simulink model "simF16_lpvplant_unmatched"  (R2020a)
settings: Solver=ode14x  StartTime=0  StopTime=sim_t  FixedStep=Ts  RelTol=1e-3  EnableMultiTasking=on
values from neighbouring files (symbols this model uses):
  adapt_gain_no_Bm = -inv(Phi)*Mat_expm    [main_f16.m]
  Ap0 = [-0.965786131048  0.940676857343; -3.44113853073  -1.30180201506]    [lpv_model.mat]    (also in parameters_twoparas_ss_large_omega_range.mat)
  Ap1 = [-0.695446741137  -0.0219021350224; -2.98749239517  -0.883673052084]    [lpv_model.mat]    (also in parameters_twoparas_ss_large_omega_range.mat)
  Ap2 = [-0.00376589285085  -0.000767161245953; 0.0864223450734  -0.00373090940113]    [lpv_model.mat]    (also in parameters_twoparas_ss_large_omega_range.mat)
  Bp0 = [-0.00202220767716 -0.26458627897]    [lpv_model.mat]    (also in parameters_twoparas_ss_large_omega_range.mat)
  Bp1 = [-0.00144075289053 -0.241352628281]    [lpv_model.mat]    (also in parameters_twoparas_ss_large_omega_range.mat)
  Bp2 = [-6.1325666296e-07 -0.000135209280723]    [lpv_model.mat]    (also in parameters_twoparas_ss_large_omega_range.mat)
  Cp = [1 0]    [lpv_model.mat]    (also in parameters_twoparas_ss_large_omega_range.mat)
  enable_L1 = 1    [main_f16.m]
  enable_um_dist_comp = 1    [main_f16.m]
  L = [-1.0529546208e-07 9.01402394984e-07 -6.3448246624e-08 3.15977865752e-07 2.28928663113e-09 -4.32057794956e-09]    [parameters_twoparas_ss_large_omega_range.mat]
  opt =     [unmatched_comp_filter.mat]
  r2d = 180/pi    (= 57.2957795131)    [main_f16.m]
  sample_time = Ts    (= 0.001)    [main_f16.m]
  Ts = 1e-3    (= 0.001)    [main_f16.m]
  unknown_input_gain = .7    (= 0.7)    [main_f16.m]
  X = [4.80336810738e-09 -1.50779531784e-08 -1.50779531784e-08 7.69063603425e-08 2.19210658353e-09 -1.15520629836e-08 -1.15520629836e-08 6.7948487849e-08 9.47019033424e-11 -1.37129742327e-10 -1.37129742327e-10 2.78905243689e-10]    [parameters_twoparas_ss_large_omega_range.mat]
undefined symbols (not defined in the file or in its folder): C_den, C_num
settings Model: ExtModeAutoUpdateStatusClock=off  Creator=keviczky  LastModifiedBy=Boran
settings DataIOCC: Decimation=50  SaveFormat=Array  SignalLoggingSaveFormat=ModelDataLogs  ReturnWorkspaceOutputs=off  SignalLoggingName=sigsOut
settings OptimizationCC: BooleanDataType=off
settings DebuggingCC: AlgebraicLoopMsg=error  SaveWithParameterizedLinksMsg=none  UnderspecifiedInitializationDetection=Classic  MergeDetectMultiDrivingBlocksExec=none  SignalResolutionControl=TryResolveAllWithWarning  MultiTaskDSMMsg=warning  MultiTaskCondExecSysMsg=none  ArithmeticOperatorsInVariantConditions=warning
settings HardwareCC: ProdBitPerPointer=32  ProdBitPerSizeT=32  ProdBitPerPtrDiffT=32  ProdLargestAtomicFloat=None  ProdIntDivRoundTo=Undefined  ProdEndianess=Unspecified  ProdWordSize=32  ProdHWDeviceType=32-bit Generic  TargetUnknown=on
settings ModelReferenceCC: PropagateSignalLabelsOutOfModel=off
settings SFSimCC: CustomCodeUndefinedFunction=UseInterfaceOnly
settings GRTTargetCC: CombineOutputUpdateFcns=off  GRTInterface=on
settings ConfigComp: CovMetricSettings=dw  CovHtmlReporting=on  CovSaveCumulativeToWorkspaceVar=on  CovSaveSingleToWorkspaceVar=on

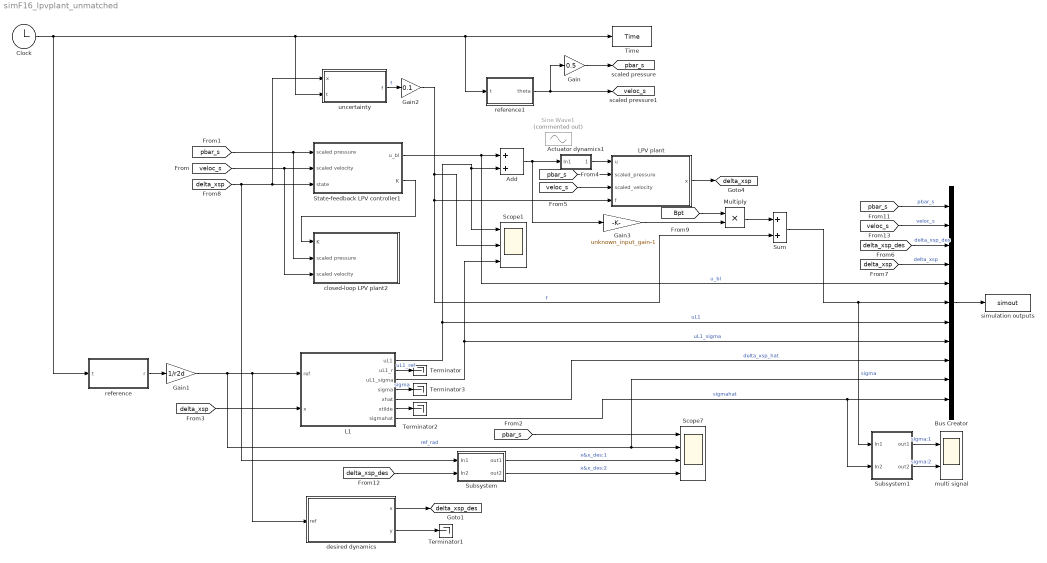
== system simF16_lpvplant_unmatched ==
  " LPV plant" : Subsystem
  Actuator dynamics1 : Subsystem
  Add : Sum
  Bus Creator : BusCreator  Inputs=11
  Clock : Clock
      settings: Decimation=50
  Gain : Gain  Gain=0.5
  Gain1 : Gain  Gain=1/r2d
  Gain2 : Gain  Gain=0.1
  Gain3 : Gain  Gain=unknown_input_gain-1
  L1 : Subsystem
  Multiply : Product
  Scope1 : Scope  NumInputPorts=3
  Scope7 : Scope  NumInputPorts=4
  Sine Wave1 : Sin  Commented=on  Frequency=2*pi*0.2  SampleTime=0
  State-feedback LPV controller1 : Subsystem
  Subsystem : Subsystem
  Subsystem1 : Subsystem
  Sum : Sum
  Terminator{,1..3} (4 alike) : Terminator
  Time : ToWorkspace  VariableName=Time  SampleTime=-1
  closed-loop LPV plant2 : Subsystem
  desired dynamics : Subsystem
  "multi signal " : Scope  NumInputPorts=2
  reference : MATLAB Function  TreatAsAtomicUnit=on
  reference1 : MATLAB Function  TreatAsAtomicUnit=on
  simulation outputs : ToWorkspace  VariableName=simout  SaveFormat=Timeseries  SampleTime=-1
  uncertainty : MATLAB Function  TreatAsAtomicUnit=on
  tag scope: delta_xsp=global, delta_xsp_des=global, pbar_s=global, veloc_s=global
  wires:
  [veloc_s] -> closed-loop LPV plant2/3(scaled velocity), State-feedback LPV controller1/2(scaled velocity)
  [pbar_s] -> closed-loop LPV plant2/2(scaled pressure), State-feedback LPV controller1/1(scaled pressure)
  State-feedback LPV controller1/2(K) -> closed-loop LPV plant2/1(K)
  State-feedback LPV controller1/1(u_bl) -> Bus Creator/5, Add/1  "u_bl"
  reference/1(r) -> Gain1/1
  Gain/1 -> [pbar_s]
  [pbar_s] -> " LPV plant"/2(scaled_pressure)
  " LPV plant"/1(x) -> [delta_xsp]
  [pbar_s] -> Scope7/1
  [delta_xsp] -> L1/2(x)
  L1/1(uL1) -> Scope1/1, Add/2, Bus Creator/7  "uL1"
  Add/1 -> Gain3/1, Actuator dynamics1/1(In1)
  Clock/1 -> reference1/1(t), Time/1, uncertainty/2(t), reference/1(t)
  L1/3(uL1_sigma) -> Scope1/3, Bus Creator/8  "uL1_sigma"
  reference1/1(theta) -> Gain/1, [veloc_s]
  [delta_xsp] -> uncertainty/1(x), State-feedback LPV controller1/3(state), Subsystem/1(In1)
  [veloc_s] -> " LPV plant"/3(scaled_velocity)
  Bus Creator/1 -> simulation outputs/1
  L1/2(uL1_r) -> Terminator/1  "uL1_ref"
  desired dynamics/1(x) -> [delta_xsp_des]
  [delta_xsp_des] -> Subsystem/2(In2)
  Subsystem/1(out1) -> Scope7/3  "x&x_des:1"
  Subsystem/2(out2) -> Scope7/4  "x&x_des:2"
  desired dynamics/2(y) -> Terminator1/1
  [pbar_s] -> Bus Creator/1  "pbar_s"
  [veloc_s] -> Bus Creator/2  "veloc_s"
  [delta_xsp_des] -> Bus Creator/3  "delta_xsp_des"
  [delta_xsp] -> Bus Creator/4  "delta_xsp"
  uncertainty/1(f) -> Gain2/1  "f"
  L1/5(xhat) -> Bus Creator/9  "delta_xsp_hat"
  Gain1/1 -> Bus Creator/10, Scope7/2, L1/1(ref), desired dynamics/1(ref)  "ref_rad"
  L1/6(xtilde) -> Terminator2/1
  Gain2/1 -> " LPV plant"/4(f), Sum/2, Scope1/2  "f"
  L1/4(sigma) -> Terminator3/1  "sigma"
  L1/7(sigmahat) -> Subsystem1/2(In2), Bus Creator/11  "sigmahat"
  [Bpt] -> Multiply/1
  Gain3/1 -> Multiply/2
  Multiply/1 -> Sum/1
  Sum/1 -> Subsystem1/1(In1), Bus Creator/6  "sigma"
  Subsystem1/1(out1) -> "multi signal "/1  "sigma:1"
  Subsystem1/2(out2) -> "multi signal "/2  "sigma:2"
  Actuator dynamics1/1(Out1) -> " LPV plant"/1(u)

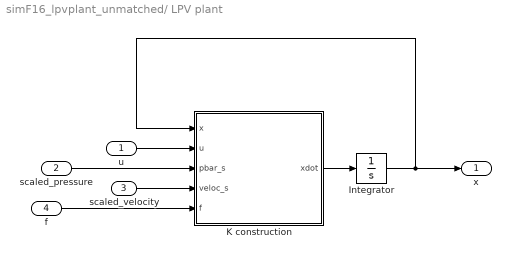
== system simF16_lpvplant_unmatched/ LPV plant ==
  u : Inport
  scaled_pressure : Inport  Port=2
  scaled_velocity : Inport  Port=3
  f : Inport  Port=4
  Integrator : Integrator
  K construction : MATLAB Function  TreatAsAtomicUnit=on
  x : Outport  VectorParamsAs1DForOutWhenUnconnected=off
  wires:
  scaled_pressure/1 -> K construction/3(pbar_s)
  u/1 -> K construction/2(u)
  K construction/1(xdot) -> Integrator/1
  Integrator/1 -> x/1, K construction/1(x)
  scaled_velocity/1 -> K construction/4(veloc_s)
  f/1 -> K construction/5(f)

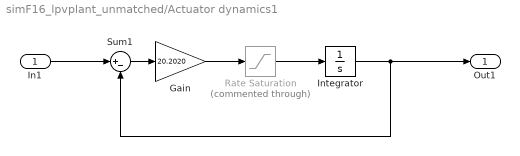
== system simF16_lpvplant_unmatched/Actuator dynamics1 ==
  In1 : Inport
  Gain : Gain  Gain=20.2020  SaturateOnIntegerOverflow=on  OutDataTypeStr=Inherit: Same as input  ParamDataTypeStr=Inherit: Same as input
  Integrator : Integrator  UpperSaturationLimit=25  LowerSaturationLimit=-25
  Rate Saturation : Saturate  Commented=through  UpperLimit=60  LowerLimit=-60
  Sum1 : Sum  Inputs=|+-  InputSameDT=on  SaturateOnIntegerOverflow=on  OutDataTypeStr=Inherit: Same as first input
  Out1 : Outport  VectorParamsAs1DForOutWhenUnconnected=off
  wires:
  Sum1/1 -> Gain/1
  Gain/1 -> Rate Saturation/1
  Integrator/1 -> Out1/1, Sum1/2
  Rate Saturation/1 -> Integrator/1
  In1/1 -> Sum1/1

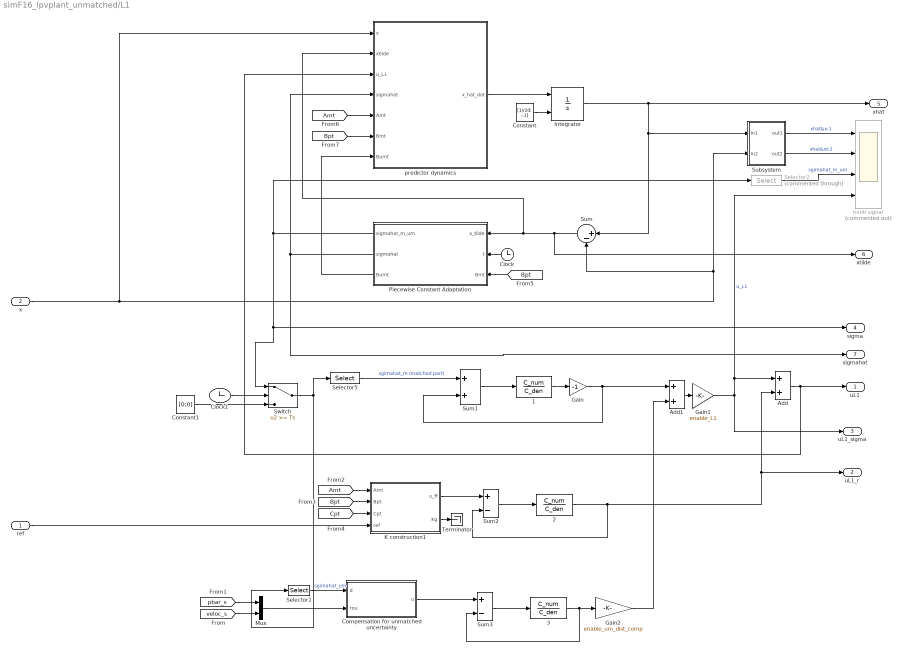
== system simF16_lpvplant_unmatched/L1 ==
  ref : Inport
  x : Inport  Port=2
  " 1" : TransferFcn  Numerator=C_num  Denominator=C_den
  " 2" : TransferFcn  Numerator=C_num  Denominator=C_den
  " 3" : TransferFcn  Numerator=C_num  Denominator=C_den
  Add : Sum
  Add1 : Sum
  Clock : Clock
  Clock1 : Clock
      settings: Decimation=50
  Compensation for unmatched uncertainty : Subsystem
  Constant : Constant  Value=[1/r2d; -.1]
  Constant1 : Constant  Value=[0;0]
  Gain : Gain  Gain=-1
  Gain1 : Gain  Gain=enable_L1
  Gain2 : Gain  Gain=enable_um_dist_comp
  Integrator : Integrator  InitialConditionSource=external
  K construction1 : MATLAB Function  TreatAsAtomicUnit=on
  Mux : Mux  Inputs=2
  Piecewise Constant Adaptation : MATLAB Function  TreatAsAtomicUnit=on
  Selector1 : Selector  InputPortWidth=2  IndexOptions=Index vector (dialog)  Indices=2  OutputSizes=1
  Selector2 : Selector  Commented=through  InputPortWidth=2  IndexOptions=Index vector (dialog)  Indices=[1]  OutputSizes=1
  Selector5 : Selector  InputPortWidth=2  IndexOptions=Index vector (dialog)  Indices=[1]  OutputSizes=1
  Subsystem : Subsystem
  Sum : Sum  Inputs=|+-
  Sum1 : Sum
  Sum2 : Sum  Inputs=+-
  Sum3 : Sum  Inputs=+-
  Switch : Switch  Threshold=Ts
  Terminator : Terminator
  "multi signal " : Scope  Commented=on  NumInputPorts=4
  predictor dynamics : MATLAB Function  TreatAsAtomicUnit=on
  uL1 : Outport  VectorParamsAs1DForOutWhenUnconnected=off
  uL1_r : Outport  Port=2  VectorParamsAs1DForOutWhenUnconnected=off
  uL1_sigma : Outport  Port=3  VectorParamsAs1DForOutWhenUnconnected=off
  sigma : Outport  Port=4  VectorParamsAs1DForOutWhenUnconnected=off
  xhat : Outport  Port=5  VectorParamsAs1DForOutWhenUnconnected=off
  xtilde : Outport  Port=6  VectorParamsAs1DForOutWhenUnconnected=off
  sigmahat : Outport  Port=7  VectorParamsAs1DForOutWhenUnconnected=off
  wires:
  Constant/1 -> Integrator/2
  predictor dynamics/1(x_hat_dot) -> Integrator/1
  Integrator/1 -> xhat/1, Sum/1, Subsystem/1(In1)
  Clock/1 -> Piecewise Constant Adaptation/2(t)
  x/1 -> Subsystem/2(In2), Sum/2, predictor dynamics/1(x)
  Piecewise Constant Adaptation/1(sigmahat_m_um) -> Switch/1, sigma/1, Selector2/1
  Selector2/1 -> "multi signal "/3  "sgimahat_m_um"
  Gain/1 -> Add1/1, Sum1/2
  " 1"/1 -> Gain/1
  [Cpt] -> K construction1/3(Cpt)
  [Bpt] -> K construction1/2(Bpt)
  ref/1 -> K construction1/4(ref)
  [Amt] -> K construction1/1(Amt)
  [Bpt] -> Piecewise Constant Adaptation/3(Bmt)
  [Amt] -> predictor dynamics/5(Amt)
  [Bpt] -> predictor dynamics/6(Bmt)
  Sum/1 -> xtilde/1, predictor dynamics/2(xtilde), Piecewise Constant Adaptation/1(x_tilde)
  Selector5/1 -> Sum1/1  "sgimahat_m (matched part)"
  Sum1/1 -> " 1"/1
  Piecewise Constant Adaptation/3(Bumt) -> predictor dynamics/7(Bumt)
  Sum2/1 -> " 2"/1
  " 2"/1 -> Sum2/2, Add/2, uL1_r/1
  Subsystem/1(out1) -> "multi signal "/1  "xhat&x:1"
  Subsystem/2(out2) -> "multi signal "/2  "xhat&xt:2"
  Add/1 -> predictor dynamics/3(u_L1), uL1/1
  K construction1/2(Kg) -> Terminator/1
  Gain1/1 -> uL1_sigma/1, Add/1, "multi signal "/4  "u_L1"
  Selector1/1 -> Compensation for unmatched uncertainty/1(d)  "sgimahat_um"
  [pbar_s] -> Mux/1
  [veloc_s] -> Mux/2
  Mux/1 -> Compensation for unmatched uncertainty/2(rou)
  " 3"/1 -> Gain2/1, Sum3/2
  Sum3/1 -> " 3"/1
  Compensation for unmatched uncertainty/1(u) -> Sum3/1
  Gain2/1 -> Add1/2
  Piecewise Constant Adaptation/2(sigmahat) -> predictor dynamics/4(sigmahat), sigmahat/1
  Add1/1 -> Gain1/1
  Switch/1 -> Selector1/1, Selector5/1
  Constant1/1 -> Switch/3
  Clock1/1 -> Switch/2
  K construction1/1(u_ff) -> Sum2/1

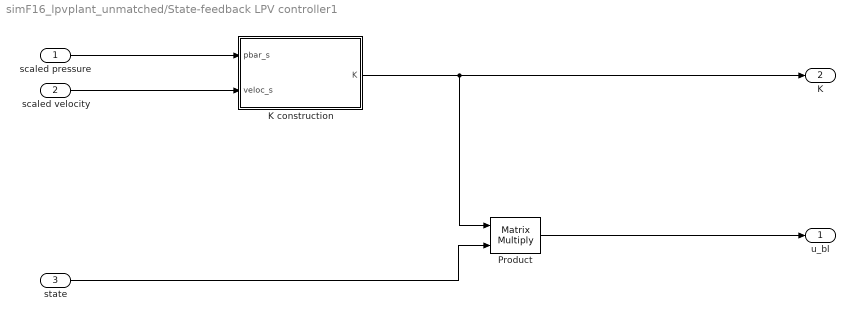
== system simF16_lpvplant_unmatched/State-feedback LPV controller1 ==
  scaled pressure : Inport
  scaled velocity : Inport  Port=2
  state : Inport  Port=3
  K construction : MATLAB Function  TreatAsAtomicUnit=on
  Product : Product  Multiplication=Matrix(*)
  u_bl : Outport  VectorParamsAs1DForOutWhenUnconnected=off
  K : Outport  Port=2  VectorParamsAs1DForOutWhenUnconnected=off
  wires:
  scaled pressure/1 -> K construction/1(pbar_s)
  K construction/1(K) -> Product/1, K/1
  state/1 -> Product/2
  Product/1 -> u_bl/1
  scaled velocity/1 -> K construction/2(veloc_s)

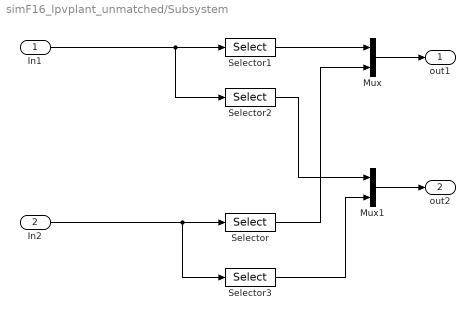
== system simF16_lpvplant_unmatched/Subsystem ==
  In1 : Inport
  In2 : Inport  Port=2
  Mux : Mux  Inputs=2
  Mux1 : Mux  Inputs=2
  Selector : Selector  InputPortWidth=2  IndexOptions=Index vector (dialog)  Indices=[1]  OutputSizes=1
  Selector1 : Selector  InputPortWidth=2  IndexOptions=Index vector (dialog)  Indices=[1]  OutputSizes=1
  Selector2 : Selector  InputPortWidth=2  IndexOptions=Index vector (dialog)  Indices=2  OutputSizes=1
  Selector3 : Selector  InputPortWidth=2  IndexOptions=Index vector (dialog)  Indices=2  OutputSizes=1
  out1 : Outport  VectorParamsAs1DForOutWhenUnconnected=off
  out2 : Outport  Port=2  VectorParamsAs1DForOutWhenUnconnected=off
  wires:
  In1/1 -> Selector2/1, Selector1/1
  In2/1 -> Selector3/1, Selector/1
  Selector/1 -> Mux/2
  Selector1/1 -> Mux/1
  Mux/1 -> out1/1
  Selector2/1 -> Mux1/1
  Selector3/1 -> Mux1/2
  Mux1/1 -> out2/1

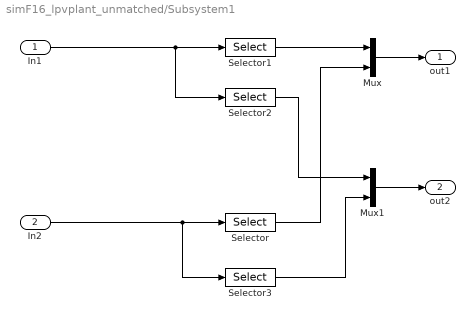
== system simF16_lpvplant_unmatched/Subsystem1 ==
  In1 : Inport
  In2 : Inport  Port=2
  Mux : Mux  Inputs=2
  Mux1 : Mux  Inputs=2
  Selector : Selector  InputPortWidth=2  IndexOptions=Index vector (dialog)  Indices=[1]  OutputSizes=1
  Selector1 : Selector  InputPortWidth=2  IndexOptions=Index vector (dialog)  Indices=[1]  OutputSizes=1
  Selector2 : Selector  InputPortWidth=2  IndexOptions=Index vector (dialog)  Indices=2  OutputSizes=1
  Selector3 : Selector  InputPortWidth=2  IndexOptions=Index vector (dialog)  Indices=2  OutputSizes=1
  out1 : Outport  VectorParamsAs1DForOutWhenUnconnected=off
  out2 : Outport  Port=2  VectorParamsAs1DForOutWhenUnconnected=off
  wires:
  In1/1 -> Selector2/1, Selector1/1
  In2/1 -> Selector3/1, Selector/1
  Selector/1 -> Mux/2
  Selector1/1 -> Mux/1
  Mux/1 -> out1/1
  Selector2/1 -> Mux1/1
  Selector3/1 -> Mux1/2
  Mux1/1 -> out2/1

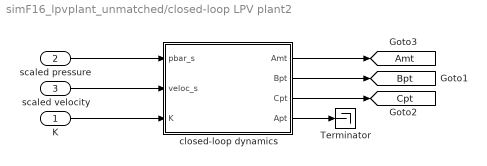
== system simF16_lpvplant_unmatched/closed-loop LPV plant2 ==
  K : Inport
  scaled pressure : Inport  Port=2
  scaled velocity : Inport  Port=3
  Terminator : Terminator
  closed-loop dynamics : MATLAB Function  TreatAsAtomicUnit=on
  tag scope: Amt=global, Bpt=global, Cpt=global
  wires:
  scaled pressure/1 -> closed-loop dynamics/1(pbar_s)
  K/1 -> closed-loop dynamics/3(K)
  closed-loop dynamics/3(Cpt) -> [Cpt]
  scaled velocity/1 -> closed-loop dynamics/2(veloc_s)
  closed-loop dynamics/1(Amt) -> [Amt]
  closed-loop dynamics/2(Bpt) -> [Bpt]
  closed-loop dynamics/4(Apt) -> Terminator/1

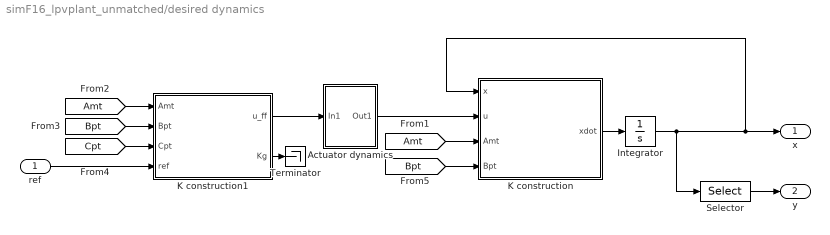
== system simF16_lpvplant_unmatched/desired dynamics ==
  ref : Inport
  Actuator dynamics : Subsystem
  Integrator : Integrator
  K construction : MATLAB Function  TreatAsAtomicUnit=on
  K construction1 : MATLAB Function  TreatAsAtomicUnit=on
  Selector : Selector  InputPortWidth=2  IndexOptions=Index vector (dialog)  Indices=1  OutputSizes=1
  Terminator : Terminator
  x : Outport  VectorParamsAs1DForOutWhenUnconnected=off
  y : Outport  Port=2  VectorParamsAs1DForOutWhenUnconnected=off
  wires:
  K construction1/2(Kg) -> Terminator/1
  [Bpt] -> K construction1/2(Bpt)
  [Amt] -> K construction1/1(Amt)
  K construction1/1(u_ff) -> Actuator dynamics/1(In1)
  ref/1 -> K construction1/4(ref)
  [Cpt] -> K construction1/3(Cpt)
  Integrator/1 -> Selector/1, x/1, K construction/1(x)
  K construction/1(xdot) -> Integrator/1
  [Amt] -> K construction/3(Amt)
  [Bpt] -> K construction/4(Bpt)
  Selector/1 -> y/1
  Actuator dynamics/1(Out1) -> K construction/2(u)

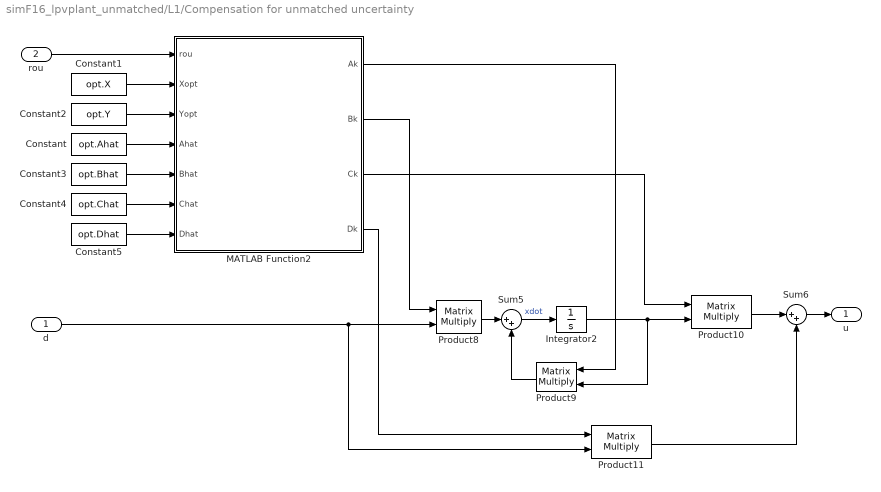
== system simF16_lpvplant_unmatched/L1/Compensation for unmatched uncertainty ==
  d : Inport
  rou : Inport  Port=2
  Constant : Constant  Value=opt.Ahat  VectorParams1D=off
  Constant1 : Constant  Value=opt.X  VectorParams1D=off
  Constant2 : Constant  Value=opt.Y  VectorParams1D=off
  Constant3 : Constant  Value=opt.Bhat  VectorParams1D=off
  Constant4 : Constant  Value=opt.Chat  VectorParams1D=off
  Constant5 : Constant  Value=opt.Dhat  VectorParams1D=off
  Integrator2 : Integrator
  MATLAB Function2 : MATLAB Function  TreatAsAtomicUnit=on
  Product{8..11} (4 alike) : Product  Multiplication=Matrix(*)
  Sum5 : Sum  Inputs=|++
  Sum6 : Sum  Inputs=|++
  u : Outport  VectorParamsAs1DForOutWhenUnconnected=off
  wires:
  d/1 -> Product8/2, Product11/2
  Sum5/1 -> Integrator2/1  "xdot"
  Product8/1 -> Sum5/1
  Product11/1 -> Sum6/2
  Product10/1 -> Sum6/1
  Integrator2/1 -> Product10/2, Product9/2
  Product9/1 -> Sum5/2
  rou/1 -> MATLAB Function2/1(rou)
  Constant/1 -> MATLAB Function2/4(Ahat)
  Sum6/1 -> u/1
  MATLAB Function2/4(Dk) -> Product11/1
  MATLAB Function2/3(Ck) -> Product10/1
  Constant4/1 -> MATLAB Function2/6(Chat)
  Constant3/1 -> MATLAB Function2/5(Bhat)
  Constant1/1 -> MATLAB Function2/2(Xopt)
  Constant2/1 -> MATLAB Function2/3(Yopt)
  MATLAB Function2/2(Bk) -> Product8/1
  Constant5/1 -> MATLAB Function2/7(Dhat)
  MATLAB Function2/1(Ak) -> Product9/1

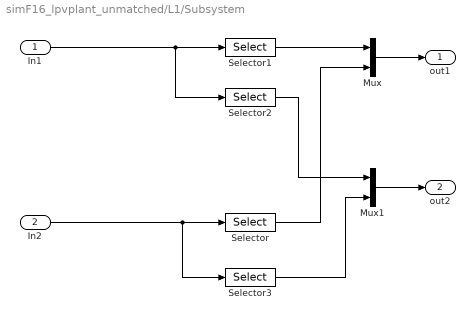
== system simF16_lpvplant_unmatched/L1/Subsystem ==
  In1 : Inport
  In2 : Inport  Port=2
  Mux : Mux  Inputs=2
  Mux1 : Mux  Inputs=2
  Selector : Selector  InputPortWidth=2  IndexOptions=Index vector (dialog)  Indices=[1]  OutputSizes=1
  Selector1 : Selector  InputPortWidth=2  IndexOptions=Index vector (dialog)  Indices=[1]  OutputSizes=1
  Selector2 : Selector  InputPortWidth=2  IndexOptions=Index vector (dialog)  Indices=2  OutputSizes=1
  Selector3 : Selector  InputPortWidth=2  IndexOptions=Index vector (dialog)  Indices=2  OutputSizes=1
  out1 : Outport  VectorParamsAs1DForOutWhenUnconnected=off
  out2 : Outport  Port=2  VectorParamsAs1DForOutWhenUnconnected=off
  wires:
  In1/1 -> Selector2/1, Selector1/1
  In2/1 -> Selector3/1, Selector/1
  Selector/1 -> Mux/2
  Selector1/1 -> Mux/1
  Mux/1 -> out1/1
  Selector2/1 -> Mux1/1
  Selector3/1 -> Mux1/2
  Mux1/1 -> out2/1

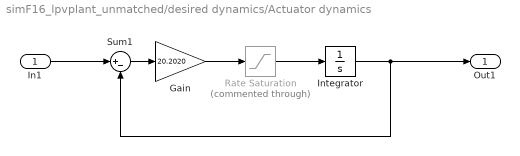
== system simF16_lpvplant_unmatched/desired dynamics/Actuator dynamics ==
  In1 : Inport
  Gain : Gain  Gain=20.2020  SaturateOnIntegerOverflow=on  OutDataTypeStr=Inherit: Same as input  ParamDataTypeStr=Inherit: Same as input
  Integrator : Integrator  UpperSaturationLimit=25  LowerSaturationLimit=-25
  Rate Saturation : Saturate  Commented=through  UpperLimit=60  LowerLimit=-60
  Sum1 : Sum  Inputs=|+-  InputSameDT=on  SaturateOnIntegerOverflow=on  OutDataTypeStr=Inherit: Same as first input
  Out1 : Outport  VectorParamsAs1DForOutWhenUnconnected=off
  wires:
  Sum1/1 -> Gain/1
  Gain/1 -> Rate Saturation/1
  Integrator/1 -> Out1/1, Sum1/2
  Rate Saturation/1 -> Integrator/1
  In1/1 -> Sum1/1

== matlab function simF16_lpvplant_unmatched/uncertainty ==
  data: x input; t input; f output
function f = fcn(x,t)
%#codegen
% f = [sin(2*pi*5*x(1))+cos(2*pi*2*t)+2*sin(2*pi*0.5*t)]; %10*x(2)^2;

% f = [0.2*sin(2*pi*10*x(1))+0.5*sin(2*pi*0.5*t); 20*x(2)*x(1)+0.5*cos(2*pi*t)]; %10*x(2)^2;

% f = [0.1*sin(2*pi*10*x(1))+0.2*sin(2*pi*0.5*t); 20*x(2)*x(1)+0.2*cos(2*pi*t)]; %10*x(2)^2; % for 100 rad/s

% f = [0.2*sin(2*pi*10*x(1))+0.2*sin(2*pi*0.5*t); 20*x(2)*x(1)+0.2*cos(2*pi*t)]; %10*x(2)^2; % for 100 rad/s

f = [0.2*sin(2*pi*10*x(1))+0.1*sin(2*pi*0.5*t); 50*x(2)*x(1)+0.1*cos(2*pi*t)]; %for nonlinear simulation

== matlab function simF16_lpvplant_unmatched/State-feedback LPV controller1/K construction ==
  data: pbar_s input; veloc_s input; X parameter; L parameter; K output
function K = CtrlConstr(pbar_s,veloc_s,X,L)
% first order polynomial
Ftheta = [1 pbar_s veloc_s];
Xt = Ftheta(1)*X(:,:,1) + Ftheta(2)*X(:,:,2) + Ftheta(3)*X(:,:,3);
Lt = Ftheta(1)*L(:,:,1) + Ftheta(2)*L(:,:,2) + Ftheta(3)*L(:,:,3);

min_eig = min(real(eig(Xt)));
if min_eig<1e-10
    disp(min_eig);
end
K = Lt/Xt;

== matlab function simF16_lpvplant_unmatched/desired dynamics/K construction ==
  data: x input; u input; Amt input; Bpt input; xdot output
function xdot  = LPV_plant(x,u,Amt,Bpt)
xdot = Amt*x+Bpt*u;

== matlab function simF16_lpvplant_unmatched/L1/predictor dynamics ==
  data: x input; xtilde input; u_L1 input; sigmahat input; x_hat_dot output size=2; Atilde parameter; Amt input; Bmt input; Bumt input
function x_hat_dot  = fcn(x, xtilde,u_L1,sigmahat, Atilde, Amt, Bmt, Bumt)

% x_hat_dot = Amt*x + Bmt*(sigmahat(1)+u_L1)+Bumt*sigmahat(2)+Atilde*xtilde; % note that the nominal input gain is an identity matrix
x_hat_dot = Amt*x + Bmt*u_L1+Atilde*xtilde+sigmahat; % note that the nominal input gain is an identity matrix

== matlab function simF16_lpvplant_unmatched/reference ==
  data: t input; r output; ref_step parameter
function r = gen_reference(t,ref_step)
%#codegen
if t<=1
    r = 0;
elseif t<=4
    r= ref_step;
else
    r = 0;
end

== matlab function simF16_lpvplant_unmatched/L1/Compensation for unmatched uncertainty/MATLAB Function2 ==
  data: rou input; Xopt input; Yopt input; Ak output; Bk output; Ck output; Dk output; Ahat input; Bhat input; Chat input; Dhat input
function [Ak,Bk,Ck,Dk] = Controller(rou,Xopt,Yopt,Ahat,Bhat,Chat,Dhat)
%#codegen
% global Khatopt Xopt Yopt 
Frou = [1 rou(1) rou(2)];
X = Xopt(:,:,1);
Y = Yopt(:,:,1);
Akhat = Ahat(:,:,1);
Bkhat = Bhat(:,:,1);
Ckhat = Chat(:,:,1);
Dkhat = Dhat(:,:,1);

for i=2:length(Frou)
    X = X + Frou(i)*Xopt(:,:,i);
    Y = Y + Frou(i)*Yopt(:,:,i);
    Akhat = Akhat + Frou(i)*Ahat(:,:,i);
    Bkhat = Bkhat + Frou(i)*Bhat(:,:,i);
    Ckhat = Ckhat + Frou(i)*Chat(:,:,i);
    Dkhat = Dkhat + Frou(i)*Dhat(:,:,i);
end

S = X-Y;
Dk = Dkhat;
Bk = Bkhat;
Ck = Ckhat/S;
Ak = Akhat/S;
if max(real(eig(Ak)))>0
   fprintf(1,'controller unstable at theta =[%.3f %.3f]',rou(1),rou(2));
end
end

== matlab function simF16_lpvplant_unmatched/reference1 ==
  settings: updateMethod=DISCRETE
  data: t input; theta output
function theta = schedule_para(t)
%#codegen
persistent theta_prev
if isempty(theta_prev)
    theta_prev = 0;    
end
if t<=10
    theta = sin(2*pi*0.2*t);   
    theta_prev = theta;
else
    theta = theta_prev;
end

== matlab function simF16_lpvplant_unmatched/closed-loop LPV plant2/closed-loop dynamics ==
  data: pbar_s input; veloc_s input; K input; Amt output; Bpt output; Cpt output; Ap0 parameter; Bp0 parameter; Ap1 parameter; Bp1 parameter; Cp parameter; Ap2 parameter; Bp2 parameter; Apt output
function [Amt,Bpt,Cpt,Apt] = LPV_plant(pbar_s,veloc_s,K,Ap0,Bp0,Ap1,Bp1,Cp,Ap2,Bp2)


Bpt = Bp0+pbar_s*Bp1+veloc_s*Bp2;
Apt = Ap0+pbar_s*Ap1+veloc_s*Ap2;
Amt = Apt+Bpt*K;
Cpt = Cp;

== matlab function simF16_lpvplant_unmatched/ LPV plant/K construction ==
  data: x input; u input; pbar_s input; veloc_s input; f input; xdot output; Ap0 parameter; Bp0 parameter; Ap1 parameter; Bp1 parameter; Cp parameter; Ap2 parameter; Bp2 parameter; unknown_input_gain parameter
function xdot   = LPV_plant(x,u,pbar_s,veloc_s,f,Ap0,Bp0,Ap1,Bp1,Cp,Ap2, Bp2,unknown_input_gain)

Bpt = Bp0+pbar_s*Bp1+veloc_s*Bp2;
Apt = Ap0+pbar_s*Ap1+veloc_s*Ap2;
Cpt = Cp;
xdot = Apt*x+Bpt*unknown_input_gain*u+f;

== matlab function simF16_lpvplant_unmatched/L1/K construction1 ==
  data: Amt input; u_ff output; Bpt input; Cpt input; ref input; Kg output
function [u_ff,Kg] = feedforward(Amt,Bpt, Cpt,ref)
Kg = -inv(Cpt/Amt*Bpt);
u_ff = Kg*ref;

== matlab function simF16_lpvplant_unmatched/L1/Piecewise Constant Adaptation ==
  settings: updateMethod=DISCRETE
  data: sigmahat_m_um output; sigmahat output; x_tilde input; t input; sample_time parameter; adapt_gain_no_Bm parameter; Bmt input; Bumt output
function [sigmahat_m_um, sigmahat,Bumt]= piecewise_constant(x_tilde,t, sample_time, adapt_gain_no_Bm,Bmt)


% Bumt = null(Bpt); %%%%%%%%%%%%% may need to hard code this to save computational time. 

Bumt = [Bmt(2);-Bmt(1)]; % to satisfy [Bmt Bumt] are full-rank and Bmt'*Bumt = 0


%%%%%%%%%%% up to here
persistent sigmahat_m_um_store;
persistent sigmahat_store;
if isempty(sigmahat_store)
    sigmahat_m_um_store = zeros(2,1);
    sigmahat_store = zeros(2,1);
end

if mod(t,sample_time) == 0   
    
    B = [Bmt Bumt];
%     adapt_gain = B\adapt_gain_no_Bm;
%        
%     sigmahat = adapt_gain*x_tilde;
    sigmahat = adapt_gain_no_Bm*x_tilde;    
    sigmahat_m_um = B\sigmahat;
    sigmahat_m_um_store = sigmahat_m_um;
    sigmahat_store = sigmahat;
else
    sigmahat_m_um = sigmahat_m_um_store;
    sigmahat = sigmahat_store;
end
% sigmahat = sigmahat(1);  % matched part

== matlab function simF16_lpvplant_unmatched/desired dynamics/K construction1 ==
  data: Amt input; u_ff output; Bpt input; Cpt input; ref input; Kg output
function [u_ff,Kg] = feedforward(Amt,Bpt, Cpt,ref)
Kg = -inv(Cpt/Amt*Bpt);
u_ff = Kg*ref;
